simulink model "cosim"
settings: Solver=FixedStepDiscrete  SolverMode=SingleTasking  StartTime=0.0  StopTime=inf  FixedStep=0.01  RelTol=1e-3
undefined symbols (not defined in the file or in its folder): A, N
libraries: xbsIndex_r4 x8, simulink x5, JTAGRuntimeCosim_r4 x1
settings Model: Creator=laca  LastModifiedBy=gaborsz
settings DataIOCC: LimitDataPoints=on  SaveFormat=Array  ReturnWorkspaceOutputs=off
settings OptimizationCC: LifeSpan=inf  SimCompilerOptimization=Off
settings DebuggingCC: UnderspecifiedInitializationDetection=Classic  MergeDetectMultiDrivingBlocksExec=none  SolverPrmCheckMsg=warning  MultiTaskDSMMsg=warning  MultiTaskCondExecSysMsg=none  FcnCallInpInsideContextMsg=Enable All  FrameProcessingCompatibilityMsg=warning  StrictBusMsg=None  SFUnexpectedBacktrackingDiag=warning  SFNoUnconditionalDefaultTransitionDiag=warning
settings HardwareCC: ProdBitPerPointer=32  ProdLargestAtomicFloat=None  ProdIntDivRoundTo=Undefined  ProdEndianess=Unspecified  ProdWordSize=32  ProdHWDeviceType=32-bit Generic
settings ModelReferenceCC: PropagateSignalLabelsOutOfModel=off
settings SFSimCC: SimUseLocalCustomCode=off
settings RTWCC: RTWUseLocalCustomCode=off  IncludeERTFirstTime=on  RTWCompilerOptimization=Off
settings CodeAppCC: CustomSymbolStrType=$N$R$M
settings GRTTargetCC: CodeReplacementLibrary=ANSI_C  GeneratePreprocessorConditionals=Disable all  CPPClassGenCompliant=off

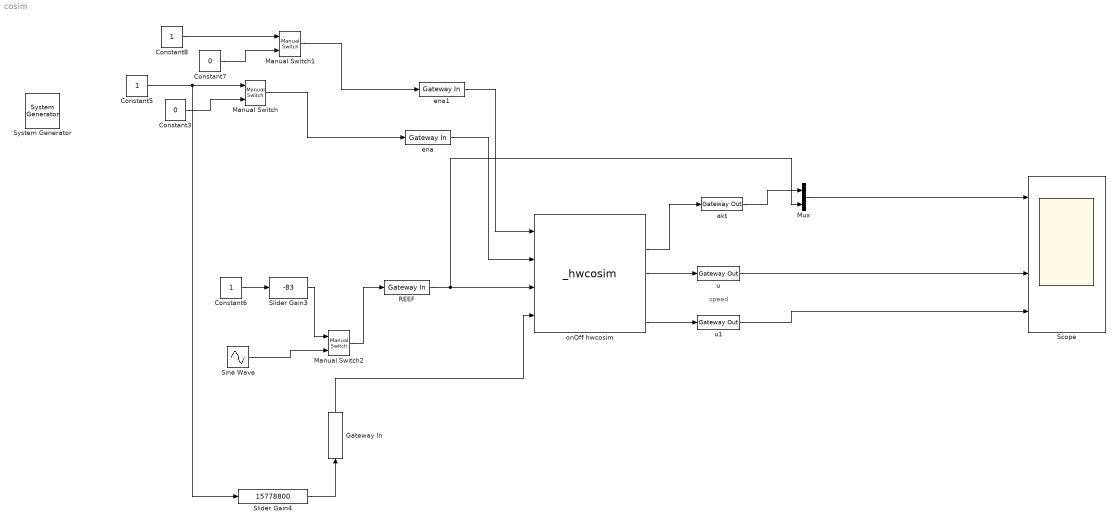
== system cosim ==
  note: speed
  " System Generator" : xbsIndex_r4/ System Generator  Tag=genX  xilinxfamily=spartan3e  part=xc3s1200e  speed=-4  package=fg320  synthesis_tool=XST  clock_wrapper=Clock Enables  directory=./netlist  proj_type=Project Navigator  Synth_file=XST Defaults  Impl_file=ISE Defaults  testbench=off  simulink_period=1  sysclk_period=20  dcm_input_clock_period=10  incr_netlist=off  trim_vbits=Everywhere in SubSystem  dbl_ovrd=According to Block Masks  core_generation=According to Block Masks  run_coregen=off  deprecated_control=off  eval_field=0  block_type=sysgen
  Constant3 : Constant  Value=0
  Constant5 : Constant
  Constant6 : Constant
  Constant7 : Constant  Value=0
  Constant8 : Constant
  Gateway In : xbsIndex_r4/Gateway In  gui_display_data_type=Fixed-point  arith_type=Unsigned  n_bits=24  bin_pt=0  preci_type=Single  exp_width=8  frac_width=24  quantization="Round  (unbiased: +/- Inf)"  overflow=Saturate  period=1  dbl_ovrd=off  timing_constraint=None  locs_specified=off  LOCs={}  UseAsADC=off  ADCChannel='1'  inherit_from_input=off  hdl_port=on  block_type=gatewayin
  Manual Switch : simulink/Signal Routing/Manual Switch  sw=0  action=0  varsize=off
  Manual Switch1 : simulink/Signal Routing/Manual Switch  sw=0  action=0  varsize=off
  Manual Switch2 : simulink/Signal Routing/Manual Switch  sw=1  action=0  varsize=off
  Mux : Mux  Inputs=2
  REEF : xbsIndex_r4/Gateway In  gui_display_data_type=Fixed-point  arith_type="Signed  (2's comp)"  n_bits=16  bin_pt=0  preci_type=Single  exp_width=8  frac_width=24  quantization="Round  (unbiased: +/- Inf)"  overflow=Saturate  period=1  dbl_ovrd=off  timing_constraint=None  locs_specified=off  LOCs={}  UseAsADC=off  ADCChannel='1'  inherit_from_input=off  hdl_port=on  block_type=gatewayin
  Scope : Scope  NumInputPorts=4
      settings: YMin=-195.3~6.65~-1~62258.3  YMax=-176.7~7.35~1~68811.8  SaveName=ScopeData2
  Sine Wave : Sin  Amplitude=90  Frequency=0.2  SampleTime=1
  Slider Gain3 : simulink/Math Operations/Slider Gain  low=-190  gain=-83  high=180
  Slider Gain4 : simulink/Math Operations/Slider Gain  low=0  gain=15778800  high=16000000
  akt : xbsIndex_r4/Gateway Out  inherit_from_input=off  hdl_port=on  timing_constraint=None  locs_specified=off  LOCs={}  UseAsDAC=off  DACChannel='1'  block_type=gatewayout
  ena : xbsIndex_r4/Gateway In  gui_display_data_type=Boolean  arith_type=Boolean  n_bits=16  bin_pt=0  preci_type=Single  exp_width=8  frac_width=24  quantization="Round  (unbiased: +/- Inf)"  overflow=Saturate  period=1  dbl_ovrd=off  timing_constraint=None  locs_specified=off  LOCs={}  UseAsADC=off  ADCChannel='1'  inherit_from_input=off  hdl_port=on  block_type=gatewayin
  ena1 : xbsIndex_r4/Gateway In  gui_display_data_type=Boolean  arith_type=Boolean  n_bits=16  bin_pt=0  preci_type=Single  exp_width=8  frac_width=24  quantization="Round  (unbiased: +/- Inf)"  overflow=Saturate  period=1  dbl_ovrd=off  timing_constraint=None  locs_specified=off  LOCs={}  UseAsADC=off  ADCChannel='1'  inherit_from_input=off  hdl_port=on  block_type=gatewayin
  onOff hwcosim : JTAGRuntimeCosim_r4/_hwcosim  clkSrc=Free Running  hasCombinationalPath=off  bitfileName=E:\Allamvizsga\Spartan3E6500SystemVer2\ONOFF\netlist\onoff_cw.bit  skipConfig=off  cable=Auto Detect  speed=N/A  cablePort=N/A  cableLocation=Local  shareCable=off  enable_codebug=on  design_xtable=|  engineDll=JTAGCosimEngine.dll  cableWaitTime=10  bscanPos=1  IRLengths=[6,8]  useWaitBox=1  hasBufgmux=on  Scheme=Cosim  useCmdProc=1  hasProc=0  useImpact=0  printLogFile=0  block_type=jtagcosim
      | {
      |   'clkWrapper' => 'onoff_cw',
      |   'clocksGcd' => undef,
      |   'device' => 'xc3s1200e-4fg320',
      |   'ports' => {
      |     'enapwm' => {
      |       'bd_port_index' => 0,
      |       'direction' => 'in',
      |       'icon_text' => 'enaPWM',
      |       'period' => 1,
      |       'sim_pause_trigger' => false,
      |       'type' => 'Bool',
      |       'width' => 1,
      |     },
      |     'ennulreset' => {
      |       'bd_port_index' => 1,
      |       'direction' => 'in',
      |       'icon_text' => 'ENnulReset',
      |       'period' => 1,
      |       'sim_pause_trigger' => false,
      |       'type' => 'Bool',
      |       'width' => 1,
      |     },
      |     'nullimp' => {
      |       'bd_port_index' => 0,
      |       'direction' => 'out',
      |       'icon_text' => 'NullImp',
      |       'period' => 1,
      |       'sim_pause_trigger' => false,
      |       'type' => 'UFix_1_0',
      |       'width' => 1,
      |     },
      |     'position' => {
      |       'bd_port_index' => 1,
      |       'direction' => 'out',
      |       'icon_text' => 'position',
      |       'period' => 1,
      |       'sim_pause_trigger' => false,
      |       'type' => 'Fix_16_0',
      |       'width' => 16,
      |     },
      |     'recerencia' => {
      |       'bd_port_index' => 2,
      |       'direction' => 'in',
      |       'icon_text' => 'recerencia',
      |       'period' => 1,
      |       'sim_pause_trigger' => false,
      |       'type' => 'Fix_16_0',
      |       'width' => 16,
      |     },
      |     'speed' => {
      |       'bd_port_index' => 2,
      |       'direction' => 'out',
      |       'icon_text' => 'speed',
      |       'period' => 1,
      |       'sim_pause_trigger' => false,
      |       'type' => 'Fix_16_0',
      |       'width' => 16,
      |     },
      |     'tsimp' => {
      |       'bd_port_index' => 3,
      |       'direction' => 'out',
      |       'icon_text' => 'Tsimp',
      |       'period' => 1,
      |       'sim_pause_trigger' => false,
      |       'type' => 'Fix_16_14',
      |       'width' => 16,
      |     },
      |     'tsvalue' => {
      |       'bd_port_index' => 3,
      |       'direction' => 'in',
      |       'icon_text' => 'TsValue',
      |       'period' => 1,
      |       'sim_pause_trigger' => false,
      |       'type' => 'UFix_24_0',
      |       'width' => 24,
      |     },
      |     'u' => {
      |       'bd_port_index' => 4,
      |       'direction' => 'out',
      |       'icon_text' => 'u',
      |       'period' => 1,
      |       'sim_pause_trigger' => false,
      |       'type' => 'Fix_17_0',
      |       'width' => 17,
      |     },
      |   },
      |   'shared_memories' => {},
      | }
  u : xbsIndex_r4/Gateway Out  inherit_from_input=off  hdl_port=on  timing_constraint=None  locs_specified=off  LOCs={}  UseAsDAC=off  DACChannel='1'  block_type=gatewayout
  u1 : xbsIndex_r4/Gateway Out  inherit_from_input=off  hdl_port=on  timing_constraint=None  locs_specified=off  LOCs={}  UseAsDAC=off  DACChannel='1'  block_type=gatewayout
  wires:
  u/1 -> Scope/3
  Manual Switch/1 -> ena/1
  Constant5/1 -> Manual Switch/1, Slider Gain4/1
  Constant3/1 -> Manual Switch/2
  Constant6/1 -> Slider Gain3/1
  Slider Gain4/1 -> Gateway In/1
  Manual Switch1/1 -> ena1/1
  Constant8/1 -> Manual Switch1/1
  Constant7/1 -> Manual Switch1/2
  u1/1 -> Scope/4
  akt/1 -> Mux/1
  Mux/1 -> Scope/1
  onOff hwcosim/5 -> u1/1
  onOff hwcosim/3 -> u/1
  onOff hwcosim/2 -> akt/1
  REEF/1 -> onOff hwcosim/3, Mux/2
  Gateway In/1 -> onOff hwcosim/4
  ena/1 -> onOff hwcosim/2
  ena1/1 -> onOff hwcosim/1
  Manual Switch2/1 -> REEF/1
  Sine Wave/1 -> Manual Switch2/2
  Slider Gain3/1 -> Manual Switch2/1
